simulink model "VTOL_renewal"  (R2023b)
settings: configuration reference "VTOLConfiguration" (kept outside this file)
undefined symbols (not defined in the file): CityMission, control, controlParams, ControlSampleTime, CriticalTiltAngle, DiscIntNeverNeededParam, env, F, FixedWingMission, flightState, FSState, FWControlParams, FWTrimSpeed, HoverMission, iniRoll, initPitch, iniYaw, Light, MIL, R_LOOKAHEAD, ReferenceFilterDen, ReferenceFilterNum, tilt_max, tilt_trim, tiltIni, TiltScheduleRate, TransitionMission, uavParam, vIni, Vt, w_trim, WindDownRate, windVel, xGround, yGround, zGround
libraries: slpidlib x56, simulink x6, uavalgslib x6, mbdriLib x4, aerolibasang x2, aerolibwind2 x2, shared6dof x1, sharedtransform x1, simulink_extras x1, sim3dlib x1, uavsim3dlib x1, uavutilslib x1
(part 8 of 8)

== system VTOL_renewal/Digital Twin/Force and Moments/Aerodynamic Forces/Compute Body Frame Forces and Moments/Wind frame F& M/Lateral Channel/Cl/roll factors ==
  p,q,r : Inport
  Airspeed : Inport  Port=2
  Constant : Constant  Value=uavParam.aero.Clp
      settings: AttributesFormatString=%<Value>
  Constant1 : Constant  Value=uavParam.aero.Clr
      settings: AttributesFormatString=%<Value>
  Get p : Selector  InputPortWidth=3  IndexOptions=Index vector (dialog)  Indices=1  OutputSizes=[(-2)]
  Get r : Selector  InputPortWidth=3  IndexOptions=Index vector (dialog)  Indices=3  OutputSizes=[(-2)]
  Product : Product  SaturateOnIntegerOverflow=on  OutDataTypeStr=Inherit: Same as first input
  Product1 : Product  SaturateOnIntegerOverflow=on  OutDataTypeStr=Inherit: Same as first input
  roll rate fact : Subsystem
  yaw rate fact : mbdriLib/Utilities/yaw rate fact  SystemSampleTime=-1  VariantActivationTime=update diagram  AllowFlexibleInterface=on  Latency=0  AutoFrameSizeCalculation=off
      link override Cmq4: Value=uavParam.geom.b
  Clp : Outport  VectorParamsAs1DForOutWhenUnconnected=off
  Clr : Outport  Port=2  VectorParamsAs1DForOutWhenUnconnected=off
  wires:
  Get r/1 -> yaw rate fact/1
  p,q,r/1 -> Get r/1, Get p/1
  Get p/1 -> roll rate fact/1(p)
  Airspeed/1 -> yaw rate fact/2, roll rate fact/2(Airspeed)
  yaw rate fact/1 -> Product1/2
  Constant1/1 -> Product1/1
  roll rate fact/1(Roll Rate Fac) -> Product/2
  Constant/1 -> Product/1
  Product1/1 -> Clr/1
  Product/1 -> Clp/1

== system VTOL_renewal/Digital Twin/Force and Moments/Aerodynamic Forces/Compute Body Frame Forces and Moments/Wind frame F& M/Lateral Channel/Cn/yaw factors ==
  p,q,r : Inport
  Airspeed : Inport  Port=2
  Constant : Constant  Value=uavParam.aero.Cnp
      settings: AttributesFormatString=%<Value>
  Constant1 : Constant  Value=uavParam.aero.Cnr
      settings: AttributesFormatString=%<Value>
  Get p : Selector  InputPortWidth=3  IndexOptions=Index vector (dialog)  Indices=1  OutputSizes=[(-2)]
  Get r : Selector  InputPortWidth=3  IndexOptions=Index vector (dialog)  Indices=3  OutputSizes=[(-2)]
  Product : Product  SaturateOnIntegerOverflow=on  OutDataTypeStr=Inherit: Same as first input
  Product1 : Product  SaturateOnIntegerOverflow=on  OutDataTypeStr=Inherit: Same as first input
  roll rate fact : Subsystem
  yaw rate fact : mbdriLib/Utilities/yaw rate fact  SystemSampleTime=-1  VariantActivationTime=update diagram  AllowFlexibleInterface=on  Latency=0  AutoFrameSizeCalculation=off
      link override Cmq4: Value=uavParam.geom.b
  Cnp : Outport  VectorParamsAs1DForOutWhenUnconnected=off
  Cnr : Outport  Port=2  VectorParamsAs1DForOutWhenUnconnected=off
  wires:
  Airspeed/1 -> yaw rate fact/2, roll rate fact/2(Airspeed)
  Get r/1 -> yaw rate fact/1
  p,q,r/1 -> Get r/1, Get p/1
  Get p/1 -> roll rate fact/1(p)
  roll rate fact/1(Roll Rate Fac) -> Product/2
  Constant/1 -> Product/1
  yaw rate fact/1 -> Product1/2
  Constant1/1 -> Product1/1
  Product1/1 -> Cnr/1
  Product/1 -> Cnp/1

== system VTOL_renewal/Digital Twin/Force and Moments/Aerodynamic Forces/Compute Body Frame Forces and Moments/Wind frame F& M/Longitudinal Channel/CL/Lift due to pitch rate ==
  p,q,r : Inport
  Airspeed : Inport  Port=2
  Constant : Constant  Value=uavParam.aero.CLq
      settings: AttributesFormatString=%<Value>
  Get q : Selector  InputPortWidth=3  IndexOptions=Index vector (dialog)  Indices=2  OutputSizes=[(-2)]
  Product : Product  SaturateOnIntegerOverflow=on  OutDataTypeStr=Inherit: Same as first input
  pitch rate factor : Subsystem
  CLq : Outport  VectorParamsAs1DForOutWhenUnconnected=off
  wires:
  Airspeed/1 -> pitch rate factor/2(Airspeed)
  Get q/1 -> pitch rate factor/1(q)
  p,q,r/1 -> Get q/1
  Product/1 -> CLq/1
  pitch rate factor/1(Pitch Rate Fac) -> Product/2
  Constant/1 -> Product/1

== system VTOL_renewal/Digital Twin/Force and Moments/Aerodynamic Forces/Compute Body Frame Forces and Moments/Wind frame F& M/Longitudinal Channel/Cm/Lift due to pitch rate ==
  p,q,r : Inport
  Airspeed : Inport  Port=2
  Constant : Constant  Value=uavParam.aero.Cmq
      settings: AttributesFormatString=%<Value>
  Get q : Selector  InputPortWidth=3  IndexOptions=Index vector (dialog)  Indices=2  OutputSizes=[(-2)]
  Product : Product  SaturateOnIntegerOverflow=on  OutDataTypeStr=Inherit: Same as first input
  pitch rate factor : Subsystem
  Cmq : Outport  VectorParamsAs1DForOutWhenUnconnected=off
  wires:
  Airspeed/1 -> pitch rate factor/2(Airspeed)
  Get q/1 -> pitch rate factor/1(q)
  p,q,r/1 -> Get q/1
  Product/1 -> Cmq/1
  pitch rate factor/1(Pitch Rate Fac) -> Product/2
  Constant/1 -> Product/1

== system VTOL_renewal/Guidance Test Bench/ControlType/Guidance Testbench/Guidance Logic/Guidance Stateflow/Guidance Mode Selector/GuidanceLogic.WP/Back Transition Guard/Triggered Subsystem ==
  Poses : Inport
  Trigger : TriggerPort  VariantControl=(inherit)
  Reshape : Reshape  OutputDimensionality=Customize  OutputDimensions=[3,1]
  Selector : Selector  InputPortWidth=4  IndexOptions=Index vector (dialog)  Indices=[1 2 3]  OutputSizes=1
  HoldPositionValue : Outport
  wires:
  Poses/1 -> Selector/1
  Selector/1 -> Reshape/1
  Reshape/1 -> HoldPositionValue/1

== system VTOL_renewal/Guidance Test Bench/ControlType/Guidance Testbench/Guidance Logic/Guidance Stateflow/Guidance Mode Selector/GuidanceLogic.WP/Dist2WP/Subsystem ==
  V : Inport
  Dot Product1 : DotProduct  OutDataTypeStr=Inherit: Inherit via internal rule
  Product : Product  Inputs=*/
  Saturation : Saturate  UpperLimit=inf  LowerLimit=0.00001
  Sqrt : Sqrt
  V_unit : Outport
  wires:
  V/1 -> Dot Product1/2, Dot Product1/1, Product/1
  Sqrt/1 -> Product/2
  Dot Product1/1 -> Saturation/1
  Saturation/1 -> Sqrt/1
  Product/1 -> V_unit/1

== system VTOL_renewal/Digital Twin/Force and Moments/Aerodynamic Forces/Compute Body Frame Forces and Moments/Wind frame F& M/Lateral Channel/CY/roll factors/Subsystem ==
  r : Inport
  Airspeed : Inport  Port=2
  Cmq3 : Constant
      settings: AttributesFormatString=%<Value>
  Cmq4 : Constant  Value=uavParam.geom.b
      settings: AttributesFormatString=%<Value>
  Gain : Gain  Gain=2
  Product1 : Product  Inputs=***/  SaturateOnIntegerOverflow=on  OutDataTypeStr=Inherit: Same as first input
  Saturation : Saturate  UpperLimit=inf  LowerLimit=0.1
      settings: AttributesFormatString="[%<LowerLimit>  %<UpperLimit>]"
  Yaw Rate Fac : Outport  VectorParamsAs1DForOutWhenUnconnected=off
  wires:
  Saturation/1 -> Gain/1
  Cmq4/1 -> Product1/3
  Airspeed/1 -> Saturation/1
  Gain/1 -> Product1/4
  Cmq3/1 -> Product1/2
  Product1/1 -> Yaw Rate Fac/1
  r/1 -> Product1/1

== system VTOL_renewal/Digital Twin/Force and Moments/Aerodynamic Forces/Compute Body Frame Forces and Moments/Wind frame F& M/Lateral Channel/CY/roll factors/roll rate fact ==
  p : Inport
  Airspeed : Inport  Port=2
  Cmq1 : Constant
      settings: AttributesFormatString=%<Value>
  Cmq2 : Constant  Value=uavParam.geom.b
      settings: AttributesFormatString=%<Value>
  Gain : Gain  Gain=2
  Product : Product  Inputs=***/  SaturateOnIntegerOverflow=on  OutDataTypeStr=Inherit: Same as first input
  Saturation : Saturate  UpperLimit=inf  LowerLimit=0.1
      settings: AttributesFormatString="[%<LowerLimit>  %<UpperLimit>]"
  Roll Rate Fac : Outport  VectorParamsAs1DForOutWhenUnconnected=off
  wires:
  Airspeed/1 -> Saturation/1
  Cmq2/1 -> Product/3
  Cmq1/1 -> Product/2
  p/1 -> Product/1
  Product/1 -> Roll Rate Fac/1
  Saturation/1 -> Gain/1
  Gain/1 -> Product/4

== system VTOL_renewal/Digital Twin/Force and Moments/Aerodynamic Forces/Compute Body Frame Forces and Moments/Wind frame F& M/Lateral Channel/Cl/roll factors/roll rate fact ==
  p : Inport
  Airspeed : Inport  Port=2
  Cmq1 : Constant  Value=.5
      settings: AttributesFormatString=%<Value>
  Cmq2 : Constant  Value=uavParam.geom.b
      settings: AttributesFormatString=%<Value>
  Product : Product  Inputs=***/  SaturateOnIntegerOverflow=on  OutDataTypeStr=Inherit: Same as first input
  Saturation : Saturate  UpperLimit=inf  LowerLimit=0.1
      settings: AttributesFormatString="[%<LowerLimit>  %<UpperLimit>]"
  Roll Rate Fac : Outport  VectorParamsAs1DForOutWhenUnconnected=off
  wires:
  Saturation/1 -> Product/4
  Airspeed/1 -> Saturation/1
  Cmq2/1 -> Product/3
  Cmq1/1 -> Product/2
  p/1 -> Product/1
  Product/1 -> Roll Rate Fac/1

== system VTOL_renewal/Digital Twin/Force and Moments/Aerodynamic Forces/Compute Body Frame Forces and Moments/Wind frame F& M/Lateral Channel/Cn/yaw factors/roll rate fact ==
  p : Inport
  Airspeed : Inport  Port=2
  Cmq1 : Constant  Value=.5
      settings: AttributesFormatString=%<Value>
  Cmq2 : Constant  Value=uavParam.geom.b
      settings: AttributesFormatString=%<Value>
  Product : Product  Inputs=***/  SaturateOnIntegerOverflow=on  OutDataTypeStr=Inherit: Same as first input
  Saturation : Saturate  UpperLimit=inf  LowerLimit=0.1
      settings: AttributesFormatString="[%<LowerLimit>  %<UpperLimit>]"
  Roll Rate Fac : Outport  VectorParamsAs1DForOutWhenUnconnected=off
  wires:
  Saturation/1 -> Product/4
  Airspeed/1 -> Saturation/1
  Cmq2/1 -> Product/3
  Cmq1/1 -> Product/2
  p/1 -> Product/1
  Product/1 -> Roll Rate Fac/1

== system VTOL_renewal/Digital Twin/Force and Moments/Aerodynamic Forces/Compute Body Frame Forces and Moments/Wind frame F& M/Longitudinal Channel/CL/Lift due to pitch rate/pitch rate factor ==
  q : Inport
  Airspeed : Inport  Port=2
  Cmq2 : Constant  Value=uavParam.geom.c
      settings: AttributesFormatString=%<Value>
  Gain : Gain  Gain=2
  Product : Product  Inputs=**/  SaturateOnIntegerOverflow=on  OutDataTypeStr=Inherit: Same as first input
  Saturation : Saturate  UpperLimit=inf  LowerLimit=0.1
      settings: AttributesFormatString="[%<LowerLimit>  %<UpperLimit>]"
  Pitch Rate Fac : Outport  VectorParamsAs1DForOutWhenUnconnected=off
  wires:
  Cmq2/1 -> Product/2
  Airspeed/1 -> Saturation/1
  q/1 -> Product/1
  Product/1 -> Pitch Rate Fac/1
  Saturation/1 -> Gain/1
  Gain/1 -> Product/3

== system VTOL_renewal/Digital Twin/Force and Moments/Aerodynamic Forces/Compute Body Frame Forces and Moments/Wind frame F& M/Longitudinal Channel/Cm/Lift due to pitch rate/pitch rate factor ==
  q : Inport
  Airspeed : Inport  Port=2
  Cmq2 : Constant  Value=uavParam.geom.c
      settings: AttributesFormatString=%<Value>
  Gain : Gain  Gain=2
  Product : Product  Inputs=**/  SaturateOnIntegerOverflow=on  OutDataTypeStr=Inherit: Same as first input
  Saturation : Saturate  UpperLimit=inf  LowerLimit=0.1
      settings: AttributesFormatString="[%<LowerLimit>  %<UpperLimit>]"
  Pitch Rate Fac : Outport  VectorParamsAs1DForOutWhenUnconnected=off
  wires:
  Cmq2/1 -> Product/2
  Airspeed/1 -> Saturation/1
  q/1 -> Product/1
  Product/1 -> Pitch Rate Fac/1
  Saturation/1 -> Gain/1
  Gain/1 -> Product/3

== matlab function VTOL_renewal/Digital Twin/Ground Truth Bus/MATLAB Function1 ==
  data: vxyz input; course output; gndSpeed output
function [course, gndSpeed] = fcn(vxyz)

vx = vxyz(1);
vy = vxyz(2);
course = atan2(vy, vx);
gndSpeed = norm([vx vy 0]);

== matlab function VTOL_renewal/Autopilot/Fixed Wing Controller/Fixed Wing Controller Simulation/Lateral Guidance Logic/MATLAB Function ==
  data: courseSP input; lacc output; course input; rollSP output; groundSpeed input; L1 input
function [lacc, rollSP] = fcn(courseSP, course, groundSpeed, L1)
eta = courseSP - course;

% wrap -pi to pi
eta = mod(eta, 2*pi);
if eta>pi
    eta = eta - 2*pi;
end

% cap eta to -pi/2 to pi/2
eta = min(eta, pi/2);
eta = max(eta, -pi/2);

lacc = 2*(groundSpeed^2)/L1*sin(eta);

rollSP = atan(lacc/9.81);

== matlab function VTOL_renewal/Autopilot/C/Attitude Controller/Pitch Roll Controller/Turn Coordinator1/MATLAB Function ==
  data: rollSP input; rSP output; pitchSP input; airSpeed input
function rSP = fcn(rollSP, pitchSP, airSpeed)
    yawRateSP = tan(rollSP)*9.81/airSpeed;
    rSP = yawRateSP*cos(pitchSP)*cos(rollSP);
end

== matlab function VTOL_renewal/Autopilot/B/Subsystem2/MATLAB Function ==
  data: phi input; y output; theta input
function y = fcn(phi,theta)

y=zeros(3,3);
y=[1 sin(phi)*tan(theta) cos(phi)*tan(theta); 0 cos(phi) -sin(phi); 0 sin(phi)/cos(theta) cos(phi)/cos(theta)];
end

== matlab function VTOL_renewal/Autopilot/C/Subsystem2/MATLAB Function ==
  data: phi input; y output; theta input
function y = fcn(phi,theta)

y=zeros(3,3);
y=[1 sin(phi)*tan(theta) cos(phi)*tan(theta); 0 cos(phi) -sin(phi); 0 sin(phi)/cos(theta) cos(phi)/cos(theta)];
end

== matlab function VTOL_renewal/Autopilot/A/Multicopter Controller/Attitude Control/Subsystem2/MATLAB Function ==
  data: phi input; y output; theta input
function y = fcn(phi,theta)

y=zeros(3,3);
y=[1 sin(phi)*tan(theta) cos(phi)*tan(theta); 0 cos(phi) -sin(phi); 0 sin(phi)/cos(theta) cos(phi)/cos(theta)];
end

== matlab function VTOL_renewal/Digital Twin/Force and Moments/Aerodynamic Drag/calcDragVector ==
  data: airVel input; dragVec output; dragCoeff input
function dragVec = fcn(airVel, dragCoeff)

dragVec = dragCoeff * norm(airVel) * airVel;

end

== matlab function VTOL_renewal/Digital Twin/Subsystem2/MATLAB Function ==
  data: phi input; y output; theta input
function y = fcn(phi,theta)

y=zeros(3,3);
y=[1 sin(phi)*tan(theta) cos(phi)*tan(theta); 0 cos(phi) -sin(phi); 0 sin(phi)/cos(theta) cos(phi)/cos(theta)];
end

== matlab function VTOL_renewal/Guidance Test Bench/ControlType/Guidance Testbench/Guidance Logic/Guidance Stateflow/Guidance Mode Selector/GuidanceLogic.BackTransition.BackTransition/MATLAB Function ==
  data: Vb input; tilt input; flag output
function flag = fcn(Vb,tilt)
tiltConditionMet=abs(tilt)<1e-1;
velocityConditionMet=abs(norm([Vb(1) 0 0]))<4;

flag=tiltConditionMet&velocityConditionMet;
end

== matlab function VTOL_renewal/Autopilot/Fixed Wing Controller/Fixed Wing Controller Simulation/Attitude Controller/Pitch Roll Controller/Turn Coordinator/MATLAB Function ==
  data: rollSP input; rSP output; pitchSP input; airSpeed input
function rSP = fcn(rollSP, pitchSP, airSpeed)
    yawRateSP = tan(rollSP)*9.81/airSpeed;
    rSP = yawRateSP*cos(pitchSP)*cos(rollSP);
end

== stateflow chart VTOL_renewal/Guidance Test Bench/ControlType/Guidance Testbench/Guidance Logic/Guidance Stateflow/Guidance Mode Selector ==
  settings: updateMethod=DISCRETE  sampleTime=UAVSampleTime*4
  state GuidanceLogic
    state FIXED_WING_WAYPOINT
      en:
      controlMode.airspeedAltitude = 1;
      controlMode.attitude = 1;
      controlMode.lateralGuidance = 1;
      state WAYPOINT
    state FIXED_WING_ENTRY
      state Stabilize
        en:
        FlightMode=flightState.FixedWing;
        controlMode.attitude = 1;
        controlMode.airspeedAltitude = 0;
        controlMode.lateralGuidance = 0;
        %Transition once done.
        FixedWingSP.yaw = 0;
        FixedWingSP.pitch = 0;
        FixedWingSP.roll = 0;
        FixedWingSP.airspeed=14;
        Status= uint8(0);
      state FIXEDWINGFLIGHT
        en:
        % Control mode
        controlMode.airspeedAltitude = 1;
        controlMode.attitude = 1;
        controlMode.lateralGuidance = 1;
        % Setpoint init
        aacSP.L1 = 25;
        aacSP.airspeed = 14;
        aacSP.altitude = 0;
        aacSP.course=0;
      (default) -> Stabilize
      Stabilize -> FIXEDWINGFLIGHT : after(3,sec)
    state Start
      en:
      %Set Flight mode to hover
      FlightMode=PresetMode;
      %Set default settings
      % Control mode
      controlMode.airspeedAltitude = 0;
      controlMode.attitude = 0;
      controlMode.lateralGuidance = 0;
      controlMode.TransitionCondition = 0;
      % Setpoint init
      FixedWingSP.yaw = 0;
      FixedWingSP.pitch = 0;
      FixedWingSP.roll = 0;
      FixedWingSP.airspeed=14;
      aacSP.L1 = 25;
      aacSP.airspeed = 14;
      aacSP.altitude = 0;
      aacSP.course=0;
      InnerLoopCmds.YawCmd=0;
    state FIXED_WING_ORBIT
      en:
      controlMode.airspeedAltitude = 1;
      controlMode.attitude = 1;
      controlMode.lateralGuidance = 1;
      state ORBIT
    state HOVER_ENTRY
      en:
      FlightMode=flightState.Hover;
      controlMode.inTransition=0;
    state Takeoff
    state WP
    state Orbit
    state PreTransition
      en:
      FlightMode=flightState.FixedWing;
      controlMode.airspeedAltitude = 1;
      controlMode.attitude = 1;
      controlMode.lateralGuidance = 1;
      % Setpoint init
      aacSP.L1 = 25;
      aacSP.airspeed = 14;
      aacSP.altitude = altitudeHold;
      aacSP.course=courseHold;
    state BackTransition
      state BackTransition
    state ForwardTransition
    state FWCOMPLETE
      Status=uint8(1);
      controlMode.TransitionCondition=uint8(1);
    note: [(mode==4)]
    state Land
      state Descend
      state WingsLevel
      state ToLand
      (default) -> ToLand
      WingsLevel -> Descend : [isLevel(States)]
      ToLand -> WingsLevel : [(norm(Pose(1:2)-ToWP.position(1:2)) <= 5)]
    (default) -> Start
    Start -> (junction 5)
    FIXEDWINGFLIGHT -> WAYPOINT [order 2] : [(mode==2)]
        | {Status=uint8(0);}
    FIXEDWINGFLIGHT -> ORBIT [order 1] : [(mode==3)]
        | {Status= uint8(0);}
    (junction 262) -> FIXED_WING_ENTRY
    (junction 5) -> FIXED_WING_ORBIT [order 6] : [(mode==3)&&(FlightMode==flightState.FixedWing)]
        | {Status=uint8(0);}
    (junction 5) -> (junction 262) [order 3] : [(FlightMode==flightState.Transition)]
        | {controlMode.inTransition=0;}
    (junction 255) -> HOVER_ENTRY
    (junction 5) -> (junction 255) [order 4] : [(FlightMode==flightState.BackTransition)]
        | {controlMode.inTransition=0;}
    HOVER_ENTRY -> (junction 12)
    (junction 257) -> FIXED_WING_WAYPOINT
    Takeoff -> WP : [Pose(3) <= ToWP.position(3)]{Status = uint8(1);}
    GuidanceLogic -> (junction 5) : [(hasChanged(mode))]
    (junction 5) -> Takeoff [order 5] : [(mode == 1)&&(FlightMode==flightState.Hover)]
        | {controlMode.inTransition=0;}
    (junction 5) -> (junction 257) [order 2] : [(mode==2)&&(FlightMode==flightState.FixedWing)]
        | {Status=uint8(0);}
    (junction 5) -> (junction 260) [order 1] : [(mode==6)&&(FlightMode==flightState.FixedWing)]
        | {courseHold=States.course;
        | altitudeHold=-States.Xe(3); }
    (junction 5) -> (junction 12) [order 7] : [FlightMode==flightState.Hover]
        | {controlMode.inTransition=0;}
    (junction 260) -> PreTransition
    (junction 12) -> WP [order 1] : [(mode==2)]
    (junction 12) -> (junction 17) [order 2]
    (junction 17) -> Orbit [order 1] : [(mode==3)]
    (junction 17) -> (junction 22) [order 2]
    PreTransition -> GuidanceLogic.BackTransition : after(5,sec)
        | {FlightMode=flightState.BackTransition;
        | controlMode.inTransition=1; }
    (junction 22) -> ForwardTransition [order 1] : [(mode==6)]
        | {FlightMode=flightState.Transition;
        | controlMode.inTransition=1;
        | controlMode.TransitionCondition=uint8(0);
        |
        | }
    (junction 22) -> Land [order 2]
    ForwardTransition -> FWCOMPLETE : [transitionConditionMet(States,Vt)]
    Land -> GuidanceLogic : [abs(Pose(3)-zGround)<=0.1]{Status = uint8(2);}
  (default) -> GuidanceLogic
  data: sf_internal_action_state_placeholder_data local double size=1 =0; sf_internal_action_state_placeholder_data local double size=1 =0; sf_internal_action_state_placeholder_data local double size=1 =0; sf_internal_action_state_placeholder_data local double size=1 =0; sf_internal_action_state_placeholder_data local double size=1 =0; sf_internal_action_state_placeholder_data local double size=1 =0; sf_internal_action_state_placeholder_data local double size=1 =0; sf_internal_action_state_placeholder_data local double size=1 =0; sf_internal_action_state_placeholder_data local double size=1 =0; sf_internal_action_state_placeholder_data local double size=1 =0; AttitudeState function_input Bus: GuidanceStates; valid function_output; TransitionSt function_input Bus: GuidanceStates; valid function_output; Vtransition function_input; mode input; ToWP input Bus: doubleUavPathManager; Status output uint8; FromWP input Bus: doubleUavPathManager; Pose input; GdncMode output Enum: GdncModeType; States input; aacSP output Bus: AAC; FixedWingSP output Bus: FixedWingCommandBus; controlMode output Bus: controlMode; FlightMode output; PresetMode input; courseHold local; altitudeHold local; Vt parameter double; InnerLoopCmds output Bus: innerLoopCmdsBus; zGround parameter
  function valid=isLevel(AttitudeState):
    | function valid=isLevel(AttitudeState)
    | %wingsLevel
    | if(norm(AttitudeState.Euler)<1e-1)&&(norm(AttitudeState.pqr)<1e-1)
    |    valid=true;
    | else
    |     valid=false;
    | end
    | 
    | end
  function valid=transitionConditionMet(TransitionSt,Vtransition):
    | function valid=transitionConditionMet(TransitionSt,Vtransition)
    | %wingsLevel
    | if(States.Tilt>=1.57)&&(vecnorm(States.Ve)>Vt)
    |    valid=true;
    | else
    |     valid=false;
    | end
    | end

== matlab function VTOL_renewal/Guidance Test Bench/ControlType/Guidance Testbench/Guidance Logic/Guidance Stateflow/Guidance Mode Selector/GuidanceLogic.Land.ToLand/MATLAB Function ==
  data: FromWP input Bus: doubleUavPathManager size=1; wps output; ToWP input Bus: doubleUavPathManager size=1
function wps = getLandingWaypoint(FromWP, ToWP)

persistent outWPS

if isempty(outWPS)
    outWPS = double(zeros(2,4));
end

outWPS(1,:) = [FromWP.position' FromWP.params(4)];
outWPS(2,:) = [ToWP.position(1:2)' FromWP.position(3) ToWP.params(4)];

wps = outWPS;

== matlab function VTOL_renewal/Guidance Test Bench/ControlType/Guidance Testbench/Guidance Logic/Guidance Stateflow/Guidance Mode Selector/GuidanceLogic.Land.WingsLevel/MATLAB Function ==
  data: FromWP input Bus: doubleUavPathManager size=1; outWPS output; ToWP input Bus: doubleUavPathManager size=1
function outWPS = getDestinationWaypoint(FromWP, ToWP)

outWPS=zeros(1,3);

outWPS(1,:) = [ToWP.position(1:2)' FromWP.position(3)];

end

== matlab function VTOL_renewal/Guidance Test Bench/ControlType/Guidance Testbench/Guidance Logic/Guidance Stateflow/Guidance Mode Selector/GuidanceLogic.WP/MATLAB Function ==
  data: FromWP input Bus: doubleUavPathManager size=1; wps output; ToWP input Bus: doubleUavPathManager size=1
function wps = getWaypointMission(FromWP, ToWP)

persistent outWPS

if isempty(outWPS)
    outWPS = double(zeros(2,4));
end

outWPS(1,:) = [FromWP.position' FromWP.params(4)];
outWPS(2,:) = [ToWP.position' ToWP.params(4)];

wps = outWPS;

== matlab function VTOL_renewal/Guidance Test Bench/ControlType/Guidance Testbench/Guidance Logic/Guidance Stateflow/Guidance Mode Selector/GuidanceLogic.FIXED_WING_WAYPOINT.WAYPOINT/MATLAB Function ==
  data: toWP input; wps output; fromWP input; alt output
function [wps, alt]= fcn(toWP, fromWP)
    wps = zeros(2,3); %#ok<PREALL> 
    wps = [fromWP'; toWP'];
    alt = -toWP(3);
end

== matlab function VTOL_renewal/Autopilot/Fixed Wing Controller/Fixed Wing Controller Simulation/Subsystem2/MATLAB Function ==
  data: phi input; y output; theta input
function y = fcn(phi,theta)

y=zeros(3,3);
y=[1 sin(phi)*tan(theta) cos(phi)*tan(theta); 0 cos(phi) -sin(phi); 0 sin(phi)/cos(theta) cos(phi)/cos(theta)];
end

== stateflow chart VTOL_renewal/Guidance Test Bench/ControlType/Manual Control/Command Interface/Basic Control  Switching ==
  state STATE_MACHINE
    state DEFAULT
      en:
      controlMode.lateralGuidance=1;
      controlMode.airspeedAltitude=1;
      controlMode.attitude=1;
      controlMode.manual=0;
      controlMode.armed=0;
      controlMode.inTransition=0;
    state TRANSITION
      controlMode.lateralGuidance=1;
      controlMode.airspeedAltitude=1;
      controlMode.attitude=1;
      controlMode.manual=0;
      controlMode.armed=0;
      controlMode.inTransition=1;
      controlMode.TransitionCondition=0;
    (default) -> DEFAULT
    STATE_MACHINE -> DEFAULT [order 2] : [hasChanged(FlightMode)]
    STATE_MACHINE -> TRANSITION [order 1] : [hasChanged(FlightMode)&&((FlightMode==flightState.Transition)||(FlightMode==flightState.BackTransition))]
    TRANSITION -> STATE_MACHINE [order 2] : [backConditioMet(States)&&(FlightMode==flightState.BackTransition)]
        | {controlMode.TransitionCondition=1;
        | controlMode.inTransition=0;}
    TRANSITION -> STATE_MACHINE [order 1] : [transitionConditionMet(States,Vt)&&(FlightMode==flightState.Transition)]
        | {controlMode.TransitionCondition=1;
        | controlMode.inTransition=0;}
  data: TransitionStates function_input Bus: GuidanceStates; valid function_output; Vtransition function_input; TransitionStates function_input Bus: GuidanceStates; valid function_output; controlMode output Bus: controlMode; FlightMode input; States input; Vt parameter double
  function valid=transitionConditionMet(TransitionStates,Vtransition):
    | function valid=transitionConditionMet(TransitionStates,Vtransition)
    | %wingsLevel
    | if((States.Tilt>=1.57)&&(vecnorm(States.Ve)>Vt))
    |    valid=true;
    | else
    |     valid=false;
    | end
    | end
  function valid=backConditioMet(TransitionStates):
    | function valid=backConditioMet(TransitionStates)
    | %wingsLevel
    | if(vecnorm(States.Ve)<1e-1)
    |    valid=true;
    | else
    |     valid=false;
    | end
    | end
